simulink model "RLS2_6_NS"  (R2024a)
settings: Solver=FixedStepAuto  StartTime=0.0  StopTime=300  FixedStep=0.3  RelTol=1e-3
libraries: dspsrcs4 x2, cstblocks x1
settings Model: Creator=mergenelos  LastModifiedBy=mergenelos

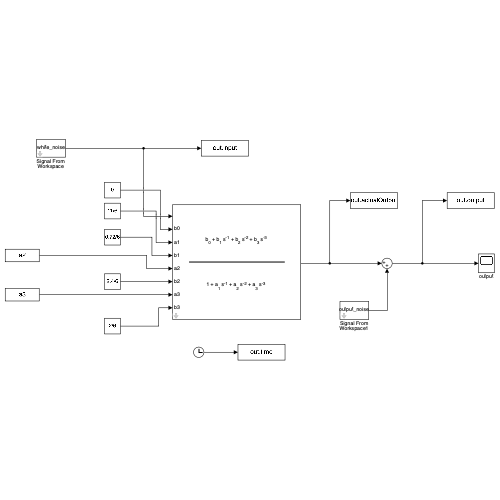
[thumbnail: Simulink's stored preview of the top-level diagram]
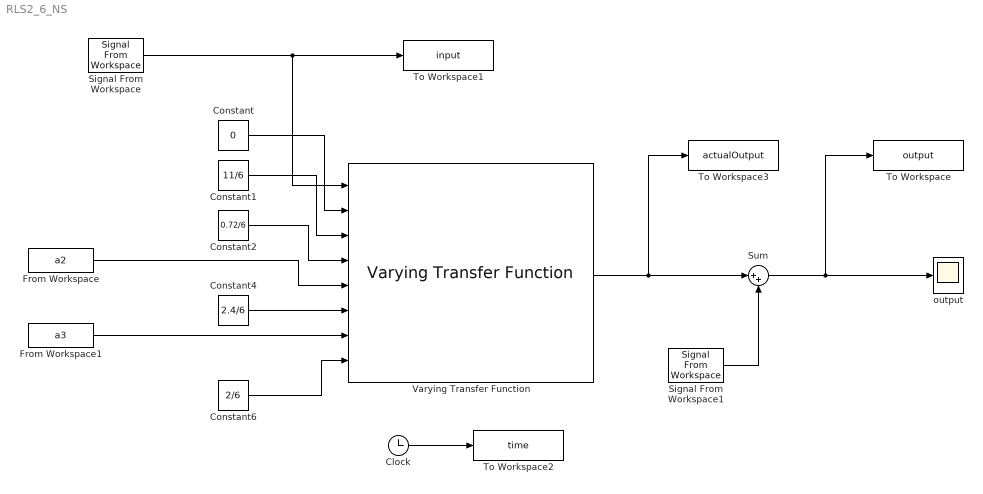
== system RLS2_6_NS ==
  Clock : Clock
  Constant : Constant  Value=0
  Constant1 : Constant  Value=11/6
  Constant2 : Constant  Value=0.72/6
  Constant4 : Constant  Value=2.4/6
  Constant6 : Constant  Value=2/6
  From Workspace : FromWorkspace  VariableName=a2  SampleTime=0.3  Interpolate=off  OutputAfterFinalValue=Holding final value
  From Workspace1 : FromWorkspace  VariableName=a3  SampleTime=0.3  Interpolate=off  OutputAfterFinalValue=Holding final value
  Signal From Workspace : dspsrcs4/Signal From Workspace  X=white_noise  Ts=0.3  nsamps=1  OutputAfterFinalValue=Setting to zero  ignoreOrWarnInputAndFrameLengths=off  OutputFrames=off
  Signal From Workspace1 : dspsrcs4/Signal From Workspace  X=output_noise  Ts=0.3  nsamps=1  OutputAfterFinalValue=Setting to zero  ignoreOrWarnInputAndFrameLengths=off  OutputFrames=off
  Sum : Sum  Inputs=|++
  To Workspace : ToWorkspace  VariableName=output  SaveFormat=Timeseries  SampleTime=-1
  To Workspace1 : ToWorkspace  VariableName=input  SaveFormat=Timeseries  SampleTime=-1
  To Workspace2 : ToWorkspace  VariableName=time  SaveFormat=Timeseries  SampleTime=-1
  To Workspace3 : ToWorkspace  VariableName=actualOutput  SaveFormat=Timeseries  SampleTime=-1
  Varying Transfer Function : cstblocks/Linear Parameter Varying/Varying Transfer Function  N=3  Feedthrough=on
  output : Scope
  wires:
  Signal From Workspace/1 -> To Workspace1/1, Varying Transfer Function/1
  Clock/1 -> To Workspace2/1
  Sum/1 -> output/1, To Workspace/1
  Signal From Workspace1/1 -> Sum/2
  Constant/1 -> Varying Transfer Function/2
  Constant1/1 -> Varying Transfer Function/3
  Constant2/1 -> Varying Transfer Function/4
  Constant4/1 -> Varying Transfer Function/6
  Constant6/1 -> Varying Transfer Function/8
  Varying Transfer Function/1 -> To Workspace3/1, Sum/1
  From Workspace/1 -> Varying Transfer Function/5
  From Workspace1/1 -> Varying Transfer Function/7
